simulink model "Mod_5_counter_stateflow"  (R2020a)
settings: Solver=FixedStepAuto  StartTime=0.0  StopTime=10  RelTol=1e-3
settings Model: Creator=Viraj  LastModifiedBy=Viraj

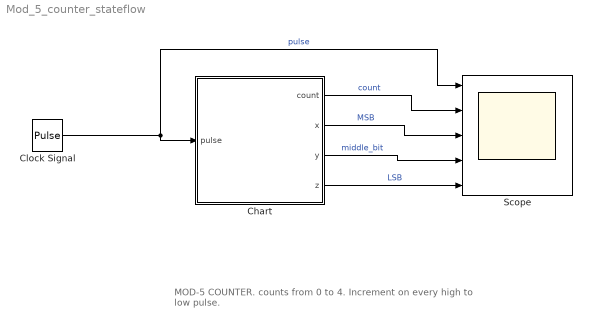
== system Mod_5_counter_stateflow ==
  note: MOD-5 COUNTER. counts from 0 to 4.
      | Increment on every high to low pulse.
  Chart : Stateflow chart  TreatAsAtomicUnit=on
  Clock Signal : DiscretePulseGenerator  PulseType=Time based  Period=1  PulseWidth=50  PhaseDelay=0.5
  Scope : Scope  NumInputPorts=5
  wires:
  Clock Signal/1 -> Scope/1, Chart/1(pulse)  "pulse"
  Chart/1(count) -> Scope/2  "count"
  Chart/2(x) -> Scope/3  "MSB"
  Chart/3(y) -> Scope/4  "middle_bit"
  Chart/4(z) -> Scope/5  "LSB"

== stateflow chart Mod_5_counter_stateflow/Chart ==
  state Binval_000_
    during:
    x = 0;
    y = 0;
    z = 0;
    count = z + y*2 + x * 4;
  state Binval_004
    during:
    x = 1;
    y = 0;
    z = 0;
    count = z + y*2 + x * 4;
  state Binval_001
    during:
    x = 0;
    y = 0;
    z = 1;
    count = z + y*2 + x * 4;
  state Binval_003
    during:
    x = 0;
    y = 1;
    z = 1;
    count = z + y*2 + x * 4;
  state Binval_002
    during:
    x = 0;
    y = 1;
    z = 0;
    count = z + y*2 + x * 4;
  (default) -> Binval_000_
  (junction 20) -> Binval_000_
  Binval_000_ -> (junction 13) : [pulse == 1]
  Binval_004 -> (junction 20) : [pulse == 1]
  (junction 13) -> Binval_001
  (junction 17) -> Binval_004 : [pulse == 1]
  Binval_001 -> (junction 15) : [pulse == 1]
  Binval_003 -> (junction 17)
  (junction 15) -> Binval_002
  Binval_002 -> Binval_003 : [pulse == 1]
  data: pulse input; count output; x output; y output; z output
